simulink model "AMdemod"  (R2021a)
settings: Solver=VariableStepAuto  StartTime=0.0  StopTime=10.0  RelTol=1e-3
libraries: hdlsllib x4, dspsrcs4 x3
settings Model: Creator=guido  LastModifiedBy=guido
settings OptimizationCC: BlockReduction=off  ConditionallyExecuteInputs=off  DefaultParameterBehavior=Inlined
settings DebuggingCC: AlgebraicLoopMsg=error
settings HardwareCC: ProdBitPerPointer=32  ProdBitPerSizeT=32  ProdBitPerPtrDiffT=32  ProdLargestAtomicFloat=None  ProdIntDivRoundTo=Undefined  ProdEndianess=Unspecified  ProdWordSize=32  ProdHWDeviceType=ASIC/FPGA->ASIC/FPGA  TargetBitPerPointer=64  TargetBitPerSizeT=64  TargetBitPerPtrDiffT=64  TargetLongLongMode=on  TargetIntDivRoundTo=Zero  TargetEndianess=LittleEndian  TargetWordSize=64  TargetHWDeviceType=Custom Processor->MATLAB Host Computer  ProdEqTarget=off

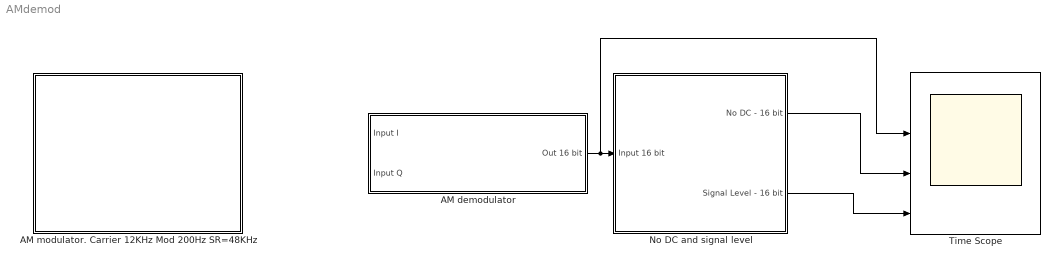
== system AMdemod ==
  AM demodulator : Subsystem
  "AM modulator. Carrier 12KHz Mod 200Hz SR=48KHz " : Subsystem
  No DC and signal level : Subsystem
  Time Scope : Scope  NumInputPorts=4
  wires:
  No DC and signal level/2("Signal Level - 16 bit ") -> Time Scope/4
  No DC and signal level/1(No DC - 16 bit) -> Time Scope/3
  ? -> Time Scope/1, AM demodulator/1(Input I)
  ? -> AM demodulator/2(Input Q)
  AM demodulator/1(Out 16 bit) -> Time Scope/2, No DC and signal level/1(Input 16 bit)

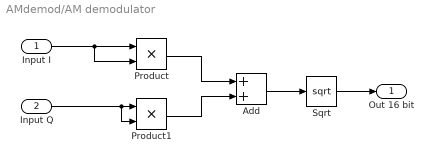
== system AMdemod/AM demodulator ==
  Input I : Inport  OutDataTypeStr=int16  SampleTime=10^-9
  Input Q : Inport  Port=2  OutDataTypeStr=int16  SampleTime=10^-9
  Add : Sum
  Product : Product  OutDataTypeStr=uint32
  Product1 : Product  OutDataTypeStr=uint32
  Sqrt : Sqrt  OutDataTypeStr=int16  SaturateOnIntegerOverflow=on
  Out 16 bit : Outport
  wires:
  Product1/1 -> Add/2
  Add/1 -> Sqrt/1
  Product/1 -> Add/1
  Input I/1 -> Product/1, Product/2
  Input Q/1 -> Product1/2, Product1/1
  Sqrt/1 -> Out 16 bit/1

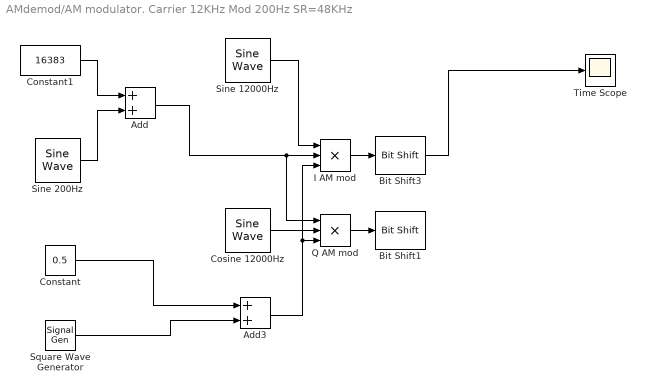
== system AMdemod/AM modulator. Carrier 12KHz Mod 200Hz SR=48KHz  ==
  Add : Sum  AccumDataTypeStr=int16  OutDataTypeStr=int16
  Add3 : Sum
  Bit Shift1 : hdlsllib/Logic and Bit Operations/Bit Shift  mode=Shift Right Arithmetic  N=16
  Bit Shift3 : hdlsllib/Logic and Bit Operations/Bit Shift  mode=Shift Right Arithmetic  N=16
  Constant : Constant  Value=0.5
  Constant1 : Constant  Value=16383  OutDataTypeStr=int16
  Cosine 12000Hz : dspsrcs4/Sine Wave  Amplitude=32767  Frequency=12000  Phase=pi/2  SampleMode=Discrete  OutComplex=Real  CompMethod=Table lookup  TableSize=Speed  SampleTime=1/48000  SamplesPerFrame=1  ResetState=Restart at time zero  OutputFrames=off  dataType=Fixed-point  wordLen=16  udDataType=sfix(16)  fracBitsMode=Best precision  numFracBits=0  OutDataTypeStr=fixdt(1,16)  LastOutDataTypeStr=fixdt(1,16)
  I AM mod : Product  Inputs=3  OutDataTypeStr=int32  SaturateOnIntegerOverflow=on
  Q AM mod : Product  Inputs=3  OutDataTypeStr=int32  SaturateOnIntegerOverflow=on
  Sine 12000Hz : dspsrcs4/Sine Wave  Amplitude=32767  Frequency=12000  Phase=0  SampleMode=Discrete  OutComplex=Real  CompMethod=Table lookup  TableSize=Speed  SampleTime=1/48000  SamplesPerFrame=1  ResetState=Restart at time zero  OutputFrames=off  dataType=Fixed-point  wordLen=16  udDataType=sfix(16)  fracBitsMode=Best precision  numFracBits=0  OutDataTypeStr=fixdt(1,16)  LastOutDataTypeStr=fixdt(1,16)
  Sine 200Hz : dspsrcs4/Sine Wave  Amplitude=16000  Frequency=800  Phase=0  SampleMode=Discrete  OutComplex=Real  CompMethod=Table lookup  TableSize=Speed  SampleTime=1/48000  SamplesPerFrame=1  ResetState=Restart at time zero  OutputFrames=off  dataType=Fixed-point  wordLen=16  udDataType=sfix(16)  fracBitsMode=Best precision  numFracBits=0  OutDataTypeStr=fixdt(1,16)  LastOutDataTypeStr=fixdt(1,16)
  Square Wave Generator : SignalGenerator  WaveForm=square  Amplitude=0.5
  Time Scope : Scope
  wires:
  Add3/1 -> I AM mod/3, Q AM mod/3
  Sine 12000Hz/1 -> I AM mod/1
  Add/1 -> Q AM mod/1, I AM mod/2
  Cosine 12000Hz/1 -> Q AM mod/2
  Constant/1 -> Add3/1
  Sine 200Hz/1 -> Add/2
  Square Wave Generator/1 -> Add3/2
  Constant1/1 -> Add/1
  I AM mod/1 -> Bit Shift3/1
  Q AM mod/1 -> Bit Shift1/1
  Bit Shift3/1 -> Time Scope/1

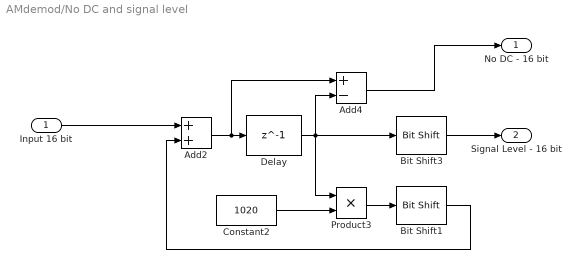
== system AMdemod/No DC and signal level ==
  Input 16 bit : Inport
  Add2 : Sum  AccumDataTypeStr=int64  OutDataTypeStr=int64
  Add4 : Sum  Inputs=+-  AccumDataTypeStr=int32  OutDataTypeStr=int16
  Bit Shift1 : hdlsllib/Logic and Bit Operations/Bit Shift  mode=Shift Right Arithmetic  N=10
  Bit Shift3 : hdlsllib/Logic and Bit Operations/Bit Shift  mode=Shift Right Arithmetic  N=9
  Constant2 : Constant  Value=1020  OutDataTypeStr=int32
  Delay : Delay  DelayLength=1  InitialCondition=1  UseCircularBuffer=on
  Product3 : Product  OutDataTypeStr=int64
  No DC - 16 bit : Outport
  "Signal Level - 16 bit " : Outport  Port=2
  wires:
  Delay/1 -> Product3/1, Bit Shift3/1, Add4/2
  Constant2/1 -> Product3/2
  Input 16 bit/1 -> Add2/1
  Add2/1 -> Add4/1, Delay/1
  Bit Shift1/1 -> Add2/2
  Bit Shift3/1 -> "Signal Level - 16 bit "/1
  Product3/1 -> Bit Shift1/1
  Add4/1 -> No DC - 16 bit/1
